simulink model "Last_version_po_STO"  (R2018b)
settings: Solver=FixedStepAuto  StartTime=0.0  StopTime=inf  FixedStep=1e-3  MaxStep=1e-4  RelTol=1e-3
undefined symbols (not defined in the file or in its folder): D11, Delta
libraries: powerlib x118, simulink_extras x25, powerlib_meascontrol x18, simulink x8, xpcutilitieslib x2, xpcrtudplib x2, opclib x1, sldrtlib x1
(part 1 of 3)
settings Model: Creator=YuORLOV  LastModifiedBy=10
settings DataIOCC: SaveOutput=off  SignalLogging=off  DSMLogging=off  SaveTime=off
settings OptimizationCC: BlockReduction=off
settings DebuggingCC: LibraryContextMissingDiagnostic=none
settings SFSimCC: SimUseLocalCustomCode=off
settings RTWCC: RTWUseLocalCustomCode=off
settings CodeAppCC: StateflowObjectComments=on
settings SimscapeCC: SimscapeNormalizeSystem=off

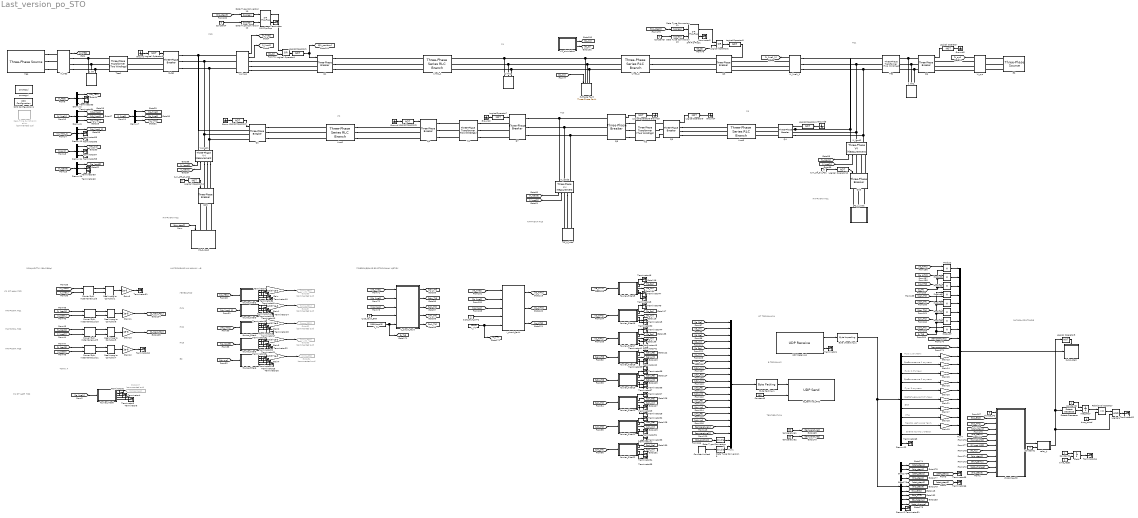
== system Last_version_po_STO ==
  note: ГЕНЕРАТОР
  note: НАПРЯЖЕНИЯ НА ШИНАХ, кВ
  note: ПС2
  note: ПС3
  note: ПС1
  note: ЭС
  note: МОЩНОСТИ, МВт(МВАр)
  note: Л1 ОТ ШИН ПС2
  note: НАГРУЗКА ПС1
  note: НАГРУЗКА ПС2
  note: НАГРУЗКА ПС3
  note: ТОКИ, А
  note: Л1 ОТ ШИН ПС2
  note: НАГРУЗКА ПС3
  note: Л2
  note: Л3
  note: ПС3
  note: ПС1
  note: ПС2
  note: НАГРУЗКА ПС1
  note: НАГРУЗКА ПС2
  note: В ТЕРМИНАЛ
  note: ПОВРЕЖДЕНИЯ ВО ВТОРИЧНЫХ ЦЕПЯХ
  note: ОТ ТЕРМИНАЛА
  note: ЗАПИСЬ COMTRADE
  note: ТЕМПЕРАТУРА
  note: Л1
  note: Пуск 1 ступени
  note: Срабатывание 1 ступени
  note: Пуск 2 ступени
  note: Срабатывание 2 ступени
  note: КТЦ
  note: Неиспр. датчиков темп.
  note: Смена группы уставок
  note: Пуск 3 ступени
  note: Срабатывание 3 ступени
  note: БНН
  1 kW : powerlib/Elements/Three-Phase Parallel RLC Load  LConnTagsString=A|B|C  Configuration=Y (grounded)  NominalVoltage=20e3  Vabc=[1e3 1e3 1e3]  Vabcp=[1e3 1e3 1e3]  NominalFrequency=50  UnbalancedPower=off  ActivePower=1000  InductivePower=0  CapacitivePower=0  Pabc=[10e3 9e3 11e3]  QLabc=[100 90 110]  QCabc=[100 90 110]  Pabcp=[10e3 9e3 11e3]  QLabcp=[100 90 110]  QCabcp=[100 90 110]  Measurements=None  LoadType=constant Z
      settings: SourceProductName=Simscape Electrical
  1 kW1 : powerlib/Elements/Three-Phase Parallel RLC Load  LConnTagsString=A|B|C  Configuration=Y (grounded)  NominalVoltage=20e3  Vabc=[1e3 1e3 1e3]  Vabcp=[1e3 1e3 1e3]  NominalFrequency=50  UnbalancedPower=off  ActivePower=1000  InductivePower=0  CapacitivePower=0  Pabc=[10e3 9e3 11e3]  QLabc=[100 90 110]  QCabc=[100 90 110]  Pabcp=[10e3 9e3 11e3]  QLabcp=[100 90 110]  QCabcp=[100 90 110]  Measurements=None  LoadType=constant Z
      settings: SourceProductName=Simscape Electrical
  1 kW2 : powerlib/Elements/Three-Phase Parallel RLC Load  LConnTagsString=A|B|C  Configuration=Y (grounded)  NominalVoltage=20e3  Vabc=[1e3 1e3 1e3]  Vabcp=[1e3 1e3 1e3]  NominalFrequency=50  UnbalancedPower=off  ActivePower=1000  InductivePower=0  CapacitivePower=0  Pabc=[10e3 9e3 11e3]  QLabc=[100 90 110]  QCabc=[100 90 110]  Pabcp=[10e3 9e3 11e3]  QLabcp=[100 90 110]  QCabcp=[100 90 110]  Measurements=None  LoadType=constant Z
      settings: SourceProductName=Simscape Electrical
  3-Phase Fault : powerlib/Elements/Three-Phase Fault  InitialStates=0  FaultA=on  FaultB=on  FaultC=off  GroundFault=on  SwitchTimes=[ 0.1 0.2]  External=on  SwitchStatus=NaN  FaultResistance=1e-3  GroundResistance=1e-3  SnubberResistance=inf  SnubberCapacitance=inf  Measurements=None
      settings: SourceProductName=Simscape Electrical
  Byte Packing 1 : xpcutilitieslib/Byte Packing   MaskPackedDataType=uint8  MaskUnpackedDataTypes={'double'}  MaskAlignment=1
  Byte Unpacking 1 : xpcutilitieslib/Byte Unpacking   MaskUnpackedDataTypes={'double'}  MaskUnpackedDataSizes={[11]}  MaskAlignment=1
      settings: SourceProductName=Simulink Real-Time  SourceProductBaseCode=XP
  Clock : Integrator  ExternalReset=either
  Constant1 : Constant  Value=4
  Constant2 : Constant
  Constant3 : Constant  Value=160  OutDataTypeStr=double
  Constant4 : Constant  Value=0
  Constant5 : Constant  Value=0
  Constant8 : Constant
  Counter Limited : simulink/Sources/Counter Limited  uplimit=3999  tsamp=-1
  Data Type Conversion{10..13} (4 alike) : DataTypeConversion  OutDataTypeStr=boolean
  Data Type Conversion8 : DataTypeConversion  OutDataTypeStr=double
  Data Type Conversion9 : DataTypeConversion  OutDataTypeStr=double
  Demux{2,6..7,10,14,16} (6 alike) : Demux  Outputs=3
  Demux22 : Demux  Outputs=11
  Demux23 : Demux  Outputs=11
  Detect Decrease : simulink/Logic and Bit Operations/Detect Decrease  vinit=0.0  OutDataTypeStr=boolean
  ES : powerlib/Electrical Sources/Three-Phase Source  InternalConnection=Y  VoltagePhases=off  Voltage=11200  PhaseAngle=0  Voltage_phases=[25e3 25e3 25e3]/sqrt(3)  PhaseAngles_phases=[0 -120 +120]  Frequency=50  NonIdealSource=on  SpecifyImpedance=on  Resistance=0.8929  Inductance=16.58e-3  ShortCircuitLevel=100e12  BaseVoltage=330e3  XRratio=999  BusType=swing  Pref=10e3  Qref=0  Prefabc=[10e3, 10e3, 10e3]  Qrefabc=[0, 0, 0]  Qmin=-inf  Qmax=inf
      settings: SourceProductName=Simscape Electrical
  Gain{,1..4} (5 alike) : Gain  Gain=sqrt(3)*1e-3
  Gain{6,10..12} (4 alike) : Gain  Gain=1e-6
  Gain{13..21} (9 alike) : Gain
  Goto107 : Goto  Commented=on  GotoTag=Irms_line1
  Goto80 : Goto  Commented=on  GotoTag=Vrms_TES
  Goto81 : Goto  Commented=on  GotoTag=Vrms_PS1
  Goto82 : Goto  Commented=on  GotoTag=Vrms_PS2
  Goto83 : Goto  Commented=on  GotoTag=Vrms_PS3
  Goto84 : Goto  Commented=on  GotoTag=Vrms_ES
  Ground{,1..7} (8 alike) : Ground
  I_circuit_fault : Subsystem
  Integrator : Integrator  ExternalReset=rising
  KZ_simulation : Subsystem
  Line1_1 : powerlib/Elements/Three-Phase Series RLC Branch  LConnTagsString=A|B|C  RConnTagsString=A|B|C  BranchType=RLC  Resistance=0.5*7.5  Inductance=0.5*120/(2*pi*50)  Capacitance=0.5*335/(2*pi*50)  Measurements=None
      settings: SourceProductName=Simscape Electrical
  Line1_2 : powerlib/Elements/Three-Phase Series RLC Branch  LConnTagsString=A|B|C  RConnTagsString=A|B|C  BranchType=RLC  Resistance=0.5*7.5  Inductance=0.5*120/(2*pi*50)  Capacitance=0.5*335/(2*pi*50)  Measurements=None
      settings: SourceProductName=Simscape Electrical
  Line2 : powerlib/Elements/Three-Phase Series RLC Branch  LConnTagsString=A|B|C  RConnTagsString=A|B|C  BranchType=RLC  Resistance=1.05  Inductance=16.25/(2*pi*50)  Capacitance=167.5/(2*pi*50)  Measurements=None
      settings: SourceProductName=Simscape Electrical
  Line3 : powerlib/Elements/Three-Phase Series RLC Branch  LConnTagsString=A|B|C  RConnTagsString=A|B|C  BranchType=RLC  Resistance=1.05  Inductance=16.25/(2*pi*50)  Capacitance=167.5/(2*pi*50)  Measurements=None
      settings: SourceProductName=Simscape Electrical
  Logical Operator{,5,11..12} (4 alike) : Logic  Operator=NOT  AllPortsSameDT=off  OutDataTypeStr=boolean
  Logical Operator1 : Logic  Operator=OR  AllPortsSameDT=off  OutDataTypeStr=boolean
  Logical Operator2 : Logic  Operator=OR  AllPortsSameDT=off  OutDataTypeStr=boolean
  Logical Operator3 : Logic  Operator=NOT  Inputs=6  AllPortsSameDT=off  OutDataTypeStr=boolean
  Logical6 : Logic  AllPortsSameDT=off  OutDataTypeStr=boolean
  LogicalOperator{1..4,6..9} (8 alike) : Logic  Operator=NOT  AllPortsSameDT=off  OutDataTypeStr=boolean
  Mux1 : Mux  Inputs=20
  Mux4 : Mux  Inputs=20
  OPC Configuration1 : opclib/OPC Configuration  errMissingItems=Error  errReadWrite=Warn  errShutdown=Error  errRTViolation=Warn  rtEnable=on  speedup=1  showLatency=off  beingUsed=on
      settings: SourceProductName=OPC Toolbox  SourceProductBaseCode=OT
  PS_1_load : Subsystem
  PS_2_load : Subsystem
  PS_3_load : Subsystem
  Power (3ph, Instantaneous){5,9..11} (4 alike) : powerlib_meascontrol/Measurements/Power (3ph, Instantaneous)
      settings: SourceProductName=Simscape Electrical
  Product{,1..7} (8 alike) : Product
  Q{1..9,25..26} (11 alike) : powerlib/Elements/Three-Phase Breaker  InitialState=closed  SwitchA=on  SwitchB=on  SwitchC=on  SwitchTimes="[1/60  5/60]"  External=on  BreakerResistance=0.01  SnubberResistance=1e6  SnubberCapacitance=inf  Measurements=None
      settings: SourceProductName=Simscape Electrical
  Q_tes : powerlib/Elements/Three-Phase Breaker  InitialState=closed  SwitchA=on  SwitchB=on  SwitchC=on  SwitchTimes="[1/60  5/60]"  External=on  BreakerResistance=0.01  SnubberResistance=1e6  SnubberCapacitance=inf  Measurements=None
      settings: SourceProductName=Simscape Electrical
  Real-Imag to Complex{1,5..7} (4 alike) : RealImagToComplex
  Real-Time Synchronization : sldrtlib/Real-Time Synchronization  Commented=on  SampleTime=0.1  MaxMissedTicks=10  ShowMissedTicks=off  YieldWhenWaiting=off
  Relational Operator : RelationalOperator  OutDataTypeStr=boolean  RndMeth=Simplest
  S-R Flip-Flop : simulink_extras/Flip Flops/S-R Flip-Flop  initial_condition=0
  S-R Flip-Flop1 : simulink_extras/Flip Flops/S-R Flip-Flop  initial_condition=0
  Subsystem : Subsystem
  TES : powerlib/Electrical Sources/Three-Phase Source  InternalConnection=Y  VoltagePhases=off  Voltage=19200  PhaseAngle=0  Voltage_phases=[25e3 25e3 25e3]/sqrt(3)  PhaseAngles_phases=[0 -120 +120]  Frequency=50  NonIdealSource=on  SpecifyImpedance=on  Resistance=0.8929  Inductance=16.58e-3  ShortCircuitLevel=100e12  BaseVoltage=330e3  XRratio=999  BusType=swing  Pref=10e3  Qref=0  Prefabc=[10e3, 10e3, 10e3]  Qrefabc=[0, 0, 0]  Qmin=-inf  Qmax=inf
      settings: SourceProductName=Simscape Electrical
  Terminator{,1..66} (67 alike) : Terminator
  Tes : powerlib/Elements/Three-Phase Transformer (Two Windings)  Winding1Connection=Yg  Winding2Connection=Delta (D11)  CoreType=Three single-phase transformers  SetSaturation=off  Hysteresis=off  DataFile='hysteresis'  SetInitialFlux=off  Measurements=None  UNITS=pu  NominalPower=[ 16500e6 , 50 ]  Winding1=[ 330e3 , 0.0005 , 0.189 ]  Winding2=[ 10.5e3 , 0.0005 , 0.189 ]  Rm=500  Lm=500  L0=0.5  Saturation=[ 0,0 ; 0.0024,1.2 ; 1.0,1.52 ]  InitialFluxes=[ 0.8 , -0.8 , 0.7 ]  MoreParameters=off  BreakLoop=off  DataType=off  TransfoNumber=1
      settings: SourceProductName=Simscape Electrical
  Tl2 : powerlib/Elements/Three-Phase Transformer (Two Windings)  Winding1Connection=Yg  Winding2Connection=Yg  CoreType=Three single-phase transformers  SetSaturation=off  Hysteresis=off  DataFile='hysteresis'  SetInitialFlux=off  Measurements=None  UNITS=pu  NominalPower=[ 100e6 , 50 ]  Winding1=[ 330e3 , 0 , 0.05 ]  Winding2=[ 110e3 , 0 , 0.05 ]  Rm=500  Lm=500  L0=0.5  Saturation=[ 0,0 ; 0.0024,1.2 ; 1.0,1.52 ]  InitialFluxes=[ 0.8 , -0.8 , 0.7 ]  MoreParameters=off  BreakLoop=off  DataType=off  TransfoNumber=1
      settings: SourceProductName=Simscape Electrical
  Tl3 : powerlib/Elements/Three-Phase Transformer (Two Windings)  Winding1Connection=Yg  Winding2Connection=Yg  CoreType=Three single-phase transformers  SetSaturation=off  Hysteresis=off  DataFile='hysteresis'  SetInitialFlux=off  Measurements=None  UNITS=pu  NominalPower=[ 100e6 , 50 ]  Winding1=[ 330e3 , 0 , 0.05 ]  Winding2=[ 110e3 , 0 , 0.05 ]  Rm=500  Lm=500  L0=0.5  Saturation=[ 0,0 ; 0.0024,1.2 ; 1.0,1.52 ]  InitialFluxes=[ 0.8 , -0.8 , 0.7 ]  MoreParameters=off  BreakLoop=off  DataType=off  TransfoNumber=1
      settings: SourceProductName=Simscape Electrical
  Ttes1 : powerlib/Elements/Three-Phase Transformer (Two Windings)  Winding1Connection=Yg  Winding2Connection=Delta (D11)  CoreType=Three single-phase transformers  SetSaturation=off  Hysteresis=off  DataFile='hysteresis'  SetInitialFlux=off  Measurements=None  UNITS=SI  NominalPower=[ 630000000, 50]  Winding1=[347000 0.19719 0.034976]  Winding2=[20000 0.00065508 0.00023238]  Rm=10029.9042  Lm=170.8631  L0=0.27511  Saturation=[0 0;3.741 1029.2;1558.8 1303.7]  InitialFluxes=[686.13 -686.13 600.37]  MoreParameters=off  BreakLoop=off  DataType=on  TransfoNumber=1
      settings: SourceProductName=Simscape Electrical
  UDP Receive1 : xpcrtudplib/UDP Receive  ipAddressVal=Use host-target connection  localPort=8002  rcvWidth=88  rcvFmAny=off  fmAddress=192.168.1.250  rcvMulticast=off  multicastAddress=[]  maxUDPQueue=8  sampleTime=1e-3
      settings: SourceProductName=Simulink Real-Time
  U_circuit_fault : Subsystem
  VI_TES : powerlib/Measurements/Three-Phase V-I Measurement  VoltageMeasurement=phase-to-ground  SetLabelV=off  LabelV=V_TES  Vpu=off  VpuLL=off  CurrentMeasurement=no  SetLabelI=off  LabelI=Iabc  Ipu=off  Pbase=100e6  Vbase=500e3  OutputType=Complex  PhasorSimulation=off  PSBequivalent=0
      settings: SourceProductName=Simscape Electrical
  VI_line1 : powerlib/Measurements/Three-Phase V-I Measurement  VoltageMeasurement=phase-to-ground  SetLabelV=off  LabelV=Vabc  Vpu=off  VpuLL=off  CurrentMeasurement=yes  SetLabelI=off  LabelI=Iabc  Ipu=off  Pbase=100e6  Vbase=500e3  OutputType=Complex  PhasorSimulation=off  PSBequivalent=0
      settings: SourceProductName=Simscape Electrical
  VI_line1_1 : powerlib/Measurements/Three-Phase V-I Measurement  VoltageMeasurement=phase-to-ground  SetLabelV=off  LabelV=Vabc  Vpu=off  VpuLL=off  CurrentMeasurement=no  SetLabelI=off  LabelI=Iabc  Ipu=off  Pbase=100e6  Vbase=500e3  OutputType=Complex  PhasorSimulation=off  PSBequivalent=0
      settings: SourceProductName=Simscape Electrical
  VI_load1 : powerlib/Measurements/Three-Phase V-I Measurement  VoltageMeasurement=phase-to-ground  SetLabelV=off  LabelV=Vabc  Vpu=off  VpuLL=off  CurrentMeasurement=yes  SetLabelI=off  LabelI=Iabc  Ipu=off  Pbase=100e6  Vbase=500e3  OutputType=Complex  PhasorSimulation=off  PSBequivalent=0
      settings: SourceProductName=Simscape Electrical
  VI_load2 : powerlib/Measurements/Three-Phase V-I Measurement  VoltageMeasurement=phase-to-ground  SetLabelV=off  LabelV=Vabc  Vpu=off  VpuLL=off  CurrentMeasurement=yes  SetLabelI=off  LabelI=Iabc  Ipu=off  Pbase=100e6  Vbase=500e3  OutputType=Complex  PhasorSimulation=off  PSBequivalent=0
      settings: SourceProductName=Simscape Electrical
  VI_load3 : powerlib/Measurements/Three-Phase V-I Measurement  VoltageMeasurement=phase-to-ground  SetLabelV=off  LabelV=Vabc  Vpu=off  VpuLL=off  CurrentMeasurement=yes  SetLabelI=off  LabelI=Iabc  Ipu=off  Pbase=100e6  Vbase=500e3  OutputType=Complex  PhasorSimulation=off  PSBequivalent=0
      settings: SourceProductName=Simscape Electrical
  VI_sys : powerlib/Measurements/Three-Phase V-I Measurement  VoltageMeasurement=phase-to-ground  SetLabelV=off  LabelV=Vabc  Vpu=off  VpuLL=off  CurrentMeasurement=no  SetLabelI=off  LabelI=Iabc  Ipu=off  Pbase=100e6  Vbase=500e3  OutputType=Complex  PhasorSimulation=off  PSBequivalent=0
      settings: SourceProductName=Simscape Electrical
  choose_PO : Constant  Value=5
  choosing_PO : Subsystem
  fourier_filter15 : Subsystem
  fourier_filter16 : Subsystem
  fourier_filter17 : Subsystem
  fourier_filter18 : Subsystem
  fourier_filter19 : Subsystem
  fourier_filter2 : Subsystem
  fourier_filter20 : Subsystem
  fourier_filter21 : Subsystem
  fourier_filter22 : Subsystem
  fourier_filter3 : Subsystem
  fourier_filter4 : Subsystem
  fourier_filter5 : Subsystem
  fourier_filter6 : Subsystem
  fourier_filter8 : Subsystem
  k_TN : Constant  Value=3300/sqrt(3)
  k_TT : Constant  Value=100/5
  powergui : powerlib/powergui  Priority=2  SimulationMode=Discrete  SampleTime=1e-3  frequency=60  Iterations=50  frequencyindice=50  Pbase=100e6  ErrMax=0.0001  UnitsV=kV  UnitsW=MW  buscounter=0  FunctionMessages=off  echomessages=off  EnableUseOfTLC=off  CurrentSourceSwitches=off  DisableSnubberDevices=off  DisableRonSwitches=off  DisableVfSwitches=off  DisplayEquations=off  SolverType=Tustin/Backward Euler (TBE)  Interpol=off  ExternalGateDelay=off  methode=off  Ts=100  x0status=blocks  SPID=off  SwTol=0  HookPort=off  RestoreLinks=warning  ResistiveCurrentMeasurement=off  Frange=logspace(0,3,50)  Ylog=off  Xlog=off  ShowGrid=off  save=off  variable=ZData  structure=0  ZoomFFT=on  StartTime=0.0  cycles=2  DisplayStyle=off  fundamental=60  FreqAxis=off  MaxFrequency=1000  frequencyindicesteady=1  RmsSteady=1  display=off
  relay_t : Subsystem
  temperature1 : Constant  Value=35  OutDataTypeStr=double
  temperature2 : Constant  Value=35  OutDataTypeStr=double
  time_cmtrd : Constant  Value=6
  time_reset : Constant
  to_terminal_RMS : xpcrtudplib/UDP Send  ipAddressVal=Use host-target connection  localPort=8001  toAddress=192.168.1.250  toPort=25001  sampleTime=1e-3
      settings: SourceProductName=Simulink Real-Time  SourceProductBaseCode=XP
  turn_off_all_PS1 : Constant  Value=0
  turn_off_all_PS2 : Constant  Value=0
  type_fault_BNN : Constant  Value=8
  type_fault_KITC : Constant
  wires:
  Logical Operator/1 -> Q6/1
  LogicalOperator1/1 -> [Q1_position], Q1/1
  LogicalOperator2/1 -> Q2/1
  LogicalOperator3/1 -> Q3/1
  LogicalOperator4/1 -> Q4/1
  VI_TES/1 -> [V_TES]
  VI_line1/2 -> [I_line1]
  VI_line1/1 -> [V_line1]
  VI_line1_1/1 -> [V_line1_1]
  VI_sys/1 -> [V_sys]
  [V_TES] -> Demux2/1
  [V_line1] -> Demux6/1
  [I_line1] -> Demux7/1
  [V_line1_1] -> Demux10/1
  [V_sys] -> Demux14/1
  Demux2/1 -> [Va_TES]
  Demux6/2 -> [Vb_line1]
  Demux6/1 -> [Va_line1]
  Demux6/3 -> [Vc_line1]
  Demux7/3 -> [Ic_line1]
  Demux7/1 -> [Ia_line1]
  Demux7/2 -> [Ib_line1]
  Demux10/1 -> [Va_line1_1]
  Demux14/1 -> [Va_sys]
  Logical Operator5/1 -> Q_tes/1
  VI_load1/1 -> [V_load2]
  VI_load1/2 -> [I_load2]
  VI_load2/2 -> [I_load1]
  VI_load2/1 -> [V_load1]
  VI_load3/1 -> [V_load3]
  VI_load3/2 -> [I_load3]
  Demux16/1 -> [Va_load3]
  [V_load3] -> Demux16/1
  [Va_TES] -> fourier_filter2/1(In1)
  [Va_line1_1] -> fourier_filter3/1(In1)
  [Va_line1] -> fourier_filter4/1(In1)
  [Va_load3] -> fourier_filter5/1(In1)
  [Va_sys] -> fourier_filter6/1(In1)
  fourier_filter2/1(RMS) -> Gain/1
  fourier_filter3/1(RMS) -> Gain1/1
  fourier_filter4/1(RMS) -> Gain2/1
  fourier_filter5/1(RMS) -> Gain3/1
  fourier_filter6/1(RMS) -> Gain4/1
  "Power (3ph, Instantaneous)5"/2 -> Real-Imag to Complex1/2
  [V_line1] -> "Power (3ph, Instantaneous)5"/1
  Real-Imag to Complex1/1 -> Gain6/1
  [I_line1] -> "Power (3ph, Instantaneous)5"/2
  "Power (3ph, Instantaneous)5"/1 -> Real-Imag to Complex1/1
  "Power (3ph, Instantaneous)9"/2 -> Real-Imag to Complex5/2
  [V_load2] -> "Power (3ph, Instantaneous)9"/1
  Real-Imag to Complex5/1 -> Gain10/1
  [I_load2] -> "Power (3ph, Instantaneous)9"/2
  "Power (3ph, Instantaneous)9"/1 -> Real-Imag to Complex5/1
  "Power (3ph, Instantaneous)10"/2 -> Real-Imag to Complex6/2
  [V_load1] -> "Power (3ph, Instantaneous)10"/1
  Real-Imag to Complex6/1 -> Gain11/1
  [I_load1] -> "Power (3ph, Instantaneous)10"/2
  "Power (3ph, Instantaneous)10"/1 -> Real-Imag to Complex6/1
  "Power (3ph, Instantaneous)11"/2 -> Real-Imag to Complex7/2
  [V_load3] -> "Power (3ph, Instantaneous)11"/1
  Real-Imag to Complex7/1 -> Gain12/1
  [I_load3] -> "Power (3ph, Instantaneous)11"/2
  "Power (3ph, Instantaneous)11"/1 -> Real-Imag to Complex7/1
  [Ia_line1] -> fourier_filter8/1(In1)
  LogicalOperator6/1 -> Q5/1
  LogicalOperator7/1 -> Q7/1
  LogicalOperator8/1 -> Q8/1
  LogicalOperator9/1 -> Q9/1
  type_fault_BNN/1 -> U_circuit_fault/4(type_fault)
  [Va_line1] -> U_circuit_fault/1(Ua)
  [Vb_line1] -> U_circuit_fault/2(Ub)
  [Vc_line1] -> U_circuit_fault/3(Uc)
  U_circuit_fault/1(U_an) -> [Uan_TN]
  U_circuit_fault/2(U_bn) -> [Ubn_TN]
  U_circuit_fault/3(U_cn) -> [Ucn_TN]
  U_circuit_fault/4(U_ni) -> [Uni_TN]
  U_circuit_fault/5(U_nk) -> [Unk_TN]
  Logical Operator11/1 -> Q25/1
  turn_off_all_PS2/1 -> Logical Operator11/1
  Logical Operator12/1 -> Q26/1
  turn_off_all_PS1/1 -> Logical Operator12/1
  KZ_simulation/1(to_KZ) -> [to_KZ]
  KZ_simulation/2(to_Q) -> [to_Q]
  [to_KZ] -> 3-Phase Fault/1
  Gain/1 -> Goto80/1
  Gain1/1 -> Goto81/1
  Gain2/1 -> Goto82/1
  Gain3/1 -> Goto83/1
  Gain4/1 -> Goto84/1
  Gain11/1 -> [S_load_PS1]
  Gain10/1 -> [S_load_PS2]
  fourier_filter8/1(RMS) -> Goto107/1
  [to_Q] -> Logical Operator1/2
  Logical Operator1/1 -> LogicalOperator1/1
  [Ia_line1] -> I_circuit_fault/1(Ia_line1)
  [Ib_line1] -> I_circuit_fault/2(Ib_line1)
  [Ic_line1] -> I_circuit_fault/3(Ic_line1)
  type_fault_KITC/1 -> I_circuit_fault/4(type_fault)
  k_TT/1 -> [k_TT], I_circuit_fault/5(k_TT)
  I_circuit_fault/1(Ia_KITC) -> [Ia_KITC]
  I_circuit_fault/3(Ic_KITC) -> [Ic_KITC]
  I_circuit_fault/2(Ib_KITC) -> [Ib_KITC]
  [Ia_KITC] -> fourier_filter15/1(In1)
  [Ib_KITC] -> fourier_filter16/1(In1)
  [Ic_KITC] -> fourier_filter17/1(In1)
  [Uan_TN] -> fourier_filter18/1(In1)
  [Ubn_TN] -> fourier_filter19/1(In1)
  [Ucn_TN] -> fourier_filter20/1(In1)
  [Uni_TN] -> fourier_filter21/1(In1)
  [Unk_TN] -> fourier_filter22/1(In1)
  fourier_filter18/2(Real) -> [Uan_Re]
  fourier_filter18/3(Imag) -> [Uan_Im]
  fourier_filter19/3(Imag) -> [Ubn_Im]
  fourier_filter19/2(Real) -> [Ubn_Re]
  fourier_filter20/3(Imag) -> [Ucn_Im]
  fourier_filter20/2(Real) -> [Ucn_Re]
  fourier_filter21/3(Imag) -> [Uni_Im]
  fourier_filter21/2(Real) -> [Uni_Re]
  fourier_filter22/3(Imag) -> [Unk_Im]
  fourier_filter22/2(Real) -> [Unk_Re]
  fourier_filter15/2(Real) -> [Ia_Re]
  fourier_filter15/3(Imag) -> [Ia_Im]
  fourier_filter16/3(Imag) -> [Ib_Im]
  fourier_filter16/2(Real) -> [Ib_Re]
  fourier_filter17/2(Real) -> [Ic_Re]
  fourier_filter17/3(Imag) -> [Ic_Im]
  [temperature1] -> Mux1/17
  [temperature2] -> Mux1/18
  [Unk_Re] -> Mux1/15
  [Unk_Im] -> Mux1/16
  [Ia_Re] -> Mux1/1
  [Uni_Im] -> Mux1/14
  [Uni_Re] -> Mux1/13
  [Ucn_Im] -> Mux1/12
  [Ucn_Re] -> Mux1/11
  [Ia_Im] -> Mux1/2
  [Ib_Re] -> Mux1/3
  [Ubn_Im] -> Mux1/10
  [Ubn_Re] -> Mux1/9
  [Uan_Im] -> Mux1/8
  [Ib_Im] -> Mux1/4
  [Uan_Re] -> Mux1/7
  [Ic_Re] -> Mux1/5
  [Ic_Im] -> Mux1/6
  Mux4/1 -> Subsystem/1(In1)
  relay_t/1(Out) -> Logical6/2, Detect Decrease/1, Logical Operator3/1
  Constant1/1 -> relay_t/2(t_vv)
  Logical Operator3/1 -> Subsystem/Enable
  k_TN/1 -> [k_TN], U_circuit_fault/5(Kt_TN)
  Product/1 -> Mux4/1
  Product1/1 -> Mux4/2
  Product2/1 -> Mux4/3
  [Ia_KITC] -> Product/1
  [Ib_KITC] -> Product1/1
  [Ic_KITC] -> Product2/1
  [k_TT] -> Product2/2, Product1/2, Product/2
  Product4/1 -> Mux4/5
  Product5/1 -> Mux4/6
  Product6/1 -> Mux4/7
  Product7/1 -> Mux4/8
  [Unk_TN] -> Product7/1
  [Uni_TN] -> Product6/1
  [Ucn_TN] -> Product5/1
  [Ubn_TN] -> Product4/1
  [Uan_TN] -> Product3/2
  [k_TN] -> Product7/2, Product6/2, Product5/2, Product4/2, Product3/1
  Constant3/1 -> to_terminal_RMS/2
  Byte Packing 1/1 -> to_terminal_RMS/1
  Mux1/1 -> Byte Packing 1/1
  UDP Receive1/1 -> Byte Unpacking 1/1
  UDP Receive1/2 -> Terminator1/1
  Byte Unpacking 1/1 -> Demux23/1, Demux22/1
  [Q1_position] -> Data Type Conversion8/1
  Data Type Conversion8/1 -> Mux1/19
  Counter Limited/1 -> Data Type Conversion9/1
  Data Type Conversion9/1 -> Mux1/20
  Product3/1 -> Mux4/4
  [temperature1] -> Mux4/9
  [temperature2] -> Mux4/10
  temperature1/1 -> [temperature1]
  temperature2/1 -> [temperature2]
  Detect Decrease/1 -> Integrator/2
  Constant8/1 -> Integrator/1
  Integrator/1 -> Relational Operator/1
  time_cmtrd/1 -> Relational Operator/2
  Relational Operator/1 -> Logical6/1
  choosing_PO/1(stop_cmtrd) -> relay_t/1(In)
  [trip_BNN] -> choosing_PO/2(trip_BNN)
  [trip_KTC] -> choosing_PO/3(trip_KTC)
  [trip_step1] -> choosing_PO/5(trip_step1)
  [sets_change] -> choosing_PO/11(sets_change)
  [fault_temp] -> choosing_PO/10(fault_temp)
  [trip_step2] -> choosing_PO/9(trip_step2)
  [start_step1] -> choosing_PO/4(start_step1)
  choose_PO/1 -> choosing_PO/1(choose_PO)
  [S_load_PS1] -> choosing_PO/6(S_load_PS1)
  [S_load_PS2] -> choosing_PO/7(S_load_PS2)
  [to_KZ] -> choosing_PO/8(to_KZ)
  Logical Operator2/1 -> LogicalOperator3/1
  [to_Q] -> Logical Operator2/2
  S-R Flip-Flop/1 -> Logical Operator1/1
  [trip_step3] -> Data Type Conversion10/1
  [trip_step3] -> Data Type Conversion11/1
  S-R Flip-Flop1/1 -> Logical Operator2/1
  Data Type Conversion10/1 -> S-R Flip-Flop/1
  Data Type Conversion11/1 -> S-R Flip-Flop1/1
  Constant4/1 -> Data Type Conversion12/1
  Data Type Conversion12/1 -> S-R Flip-Flop/2
  Constant5/1 -> Data Type Conversion13/1
  Data Type Conversion13/1 -> S-R Flip-Flop1/2
  S-R Flip-Flop/2 -> Terminator/1
  S-R Flip-Flop1/2 -> Terminator2/1
  fourier_filter8/2(Real) -> Terminator3/1
  fourier_filter8/3(Imag) -> Terminator4/1
  fourier_filter8/4(Complex) -> Terminator5/1
  fourier_filter8/5(Phase) -> Terminator6/1
  fourier_filter2/2(Real) -> Terminator7/1
  fourier_filter2/3(Imag) -> Terminator8/1
  fourier_filter2/5(Phase) -> Terminator10/1
  fourier_filter2/4(Complex) -> Terminator9/1
  fourier_filter3/2(Real) -> Terminator11/1
  fourier_filter3/3(Imag) -> Terminator12/1
  fourier_filter3/4(Complex) -> Terminator13/1
  fourier_filter3/5(Phase) -> Terminator14/1
  fourier_filter4/2(Real) -> Terminator15/1
  fourier_filter4/3(Imag) -> Terminator16/1
  fourier_filter4/4(Complex) -> Terminator17/1
  fourier_filter4/5(Phase) -> Terminator18/1
  fourier_filter5/2(Real) -> Terminator19/1
  fourier_filter5/3(Imag) -> Terminator20/1
  fourier_filter5/4(Complex) -> Terminator21/1
  fourier_filter5/5(Phase) -> Terminator22/1
  fourier_filter6/2(Real) -> Terminator23/1
  fourier_filter6/3(Imag) -> Terminator24/1
  fourier_filter6/4(Complex) -> Terminator25/1
  fourier_filter6/5(Phase) -> Terminator26/1
  fourier_filter20/1(RMS) -> Terminator27/1
  fourier_filter20/5(Phase) -> Terminator28/1
  fourier_filter20/4(Complex) -> Terminator29/1
  fourier_filter21/4(Complex) -> Terminator31/1
  fourier_filter21/5(Phase) -> Terminator30/1
  fourier_filter21/1(RMS) -> Terminator32/1
  fourier_filter22/1(RMS) -> Terminator33/1
  fourier_filter22/4(Complex) -> Terminator34/1
  fourier_filter22/5(Phase) -> Terminator35/1
  fourier_filter19/5(Phase) -> Terminator36/1
  fourier_filter19/4(Complex) -> Terminator37/1
  fourier_filter19/1(RMS) -> Terminator38/1
  fourier_filter18/5(Phase) -> Terminator39/1
  fourier_filter18/4(Complex) -> Terminator40/1
  fourier_filter18/1(RMS) -> Terminator41/1
  fourier_filter17/5(Phase) -> Terminator42/1
  fourier_filter17/4(Complex) -> Terminator43/1
  fourier_filter17/1(RMS) -> Terminator44/1
  fourier_filter16/5(Phase) -> Terminator45/1
  fourier_filter15/1(RMS) -> Terminator46/1
  fourier_filter15/4(Complex) -> Terminator47/1
  fourier_filter15/5(Phase) -> Terminator48/1
  fourier_filter16/1(RMS) -> Terminator49/1
  fourier_filter16/4(Complex) -> Terminator50/1
  Ground/1 -> LogicalOperator2/1
  Ground1/1 -> LogicalOperator6/1
  Ground2/1 -> LogicalOperator7/1
  Ground3/1 -> LogicalOperator8/1
  Ground4/1 -> LogicalOperator9/1
  Ground5/1 -> LogicalOperator4/1
  Ground6/1 -> Logical Operator/1
  Ground7/1 -> Logical Operator5/1
  Logical6/1 -> Terminator52/1
  Demux2/2 -> Terminator53/1
  Demux2/3 -> Terminator54/1
  Demux10/2 -> Terminator55/1
  Demux10/3 -> Terminator56/1
  Demux14/2 -> Terminator57/1
  Demux14/3 -> Terminator58/1
  Demux16/2 -> Terminator59/1
  Demux16/3 -> Terminator60/1
  Gain6/1 -> Terminator61/1
  Gain12/1 -> Terminator62/1
  Gain21/1 -> Mux4/16
  Gain20/1 -> Mux4/15
  Gain17/1 -> Mux4/17
  Gain19/1 -> Mux4/19
  Gain18/1 -> Mux4/18
  Gain16/1 -> Mux4/14
  Gain15/1 -> Mux4/13
  Gain14/1 -> Mux4/12
  Gain13/1 -> Mux4/11
  Demux22/2 -> Gain14/1
  Demux22/1 -> Gain13/1
  Demux22/3 -> Gain15/1
  Demux22/4 -> Gain16/1
  Demux22/5 -> Gain20/1
  Demux22/6 -> Gain21/1
  Demux22/7 -> Gain17/1
  Demux22/8 -> Gain18/1
  Demux22/9 -> Gain19/1
  Demux22/10 -> Mux4/20
  Demux23/6 -> [trip_step3]
  Demux23/5 -> [start_step3]
  Demux23/4 -> [trip_step2]
  Demux23/10 -> [sets_change]
  Demux23/9 -> [fault_temp]
  Demux23/8 -> [trip_KTC]
  Demux23/7 -> [trip_BNN]
  Demux23/3 -> [start_step2]
  Demux23/2 -> [trip_step1]
  Demux23/1 -> [start_step1]
  Demux23/11 -> Terminator51/1
  [trip_step2] -> PS_2_load/1(trip_step2)
  [trip_step3] -> choosing_PO/12(trip_step3)
  Constant2/1 -> Clock/1
  time_reset/1 -> Clock/2
  Demux22/11 -> Terminator63/1
  Clock/1 -> Terminator64/1
  [start_step2] -> Terminator65/1
  [start_step3] -> Terminator66/1
  connections:
  Line1_2/LConn1 -- 1 kW1/LConn1 -- Line1_1/RConn1 -- 3-Phase Fault/LConn1
  Line1_2/LConn2 -- 1 kW1/LConn2 -- Line1_1/RConn2 -- 3-Phase Fault/LConn2
  Line1_2/LConn3 -- 1 kW1/LConn3 -- Line1_1/RConn3 -- 3-Phase Fault/LConn3
  Tes/LConn3 -- VI_load2/LConn3 -- Q4/LConn3 -- VI_line1_1/LConn3
  Q6/RConn1 -- 1 kW2/LConn1 -- Tes/RConn1
  Q6/RConn2 -- 1 kW2/LConn2 -- Tes/RConn2
  Q6/RConn3 -- 1 kW2/LConn3 -- Tes/RConn3
  VI_sys/RConn3 -- Q6/LConn3
  VI_sys/RConn2 -- Q6/LConn2
  VI_sys/RConn1 -- Q6/LConn1
  ES/RConn1 -- VI_sys/LConn1
  ES/RConn2 -- VI_sys/LConn2
  ES/RConn3 -- VI_sys/LConn3
  Q1/RConn1 -- Line1_1/LConn1
  Q1/RConn2 -- Line1_1/LConn2
  Q1/RConn3 -- Line1_1/LConn3
  Q2/RConn1 -- Line2/LConn1
  Q2/RConn2 -- Line2/LConn2
  Q2/RConn3 -- Line2/LConn3
  Q3/RConn1 -- Line1_2/RConn1
  Q3/RConn3 -- Line1_2/RConn3
  Q4/RConn1 -- Line3/RConn1
  Q4/RConn2 -- Line3/RConn2
  Q4/RConn3 -- Line3/RConn3
  VI_line1/RConn2 -- Q1/LConn2
  VI_line1/RConn1 -- Q1/LConn1
  VI_line1/RConn3 -- Q1/LConn3
  Line1_2/RConn2 -- Q3/RConn2
  Q_tes/LConn1 -- Ttes1/LConn1
  Q_tes/LConn2 -- Ttes1/LConn2
  Q_tes/LConn3 -- Ttes1/LConn3
  VI_line1/LConn2 -- VI_load1/LConn2 -- Q2/LConn2 -- Q_tes/RConn2
  Q_tes/RConn1 -- VI_load1/LConn1 -- Q2/LConn1 -- VI_line1/LConn1
  VI_line1_1/RConn2 -- Q3/LConn2
  VI_line1_1/RConn1 -- Q3/LConn1
  VI_line1_1/RConn3 -- Q3/LConn3
  Tes/LConn2 -- VI_load2/LConn2 -- Q4/LConn2 -- VI_line1_1/LConn2
  Q4/LConn1 -- VI_line1_1/LConn1 -- Tes/LConn1 -- VI_load2/LConn1
  VI_line1/LConn3 -- VI_load1/LConn3 -- Q2/LConn3 -- Q_tes/RConn3
  VI_load1/RConn2 -- Q25/LConn2
  Q5/RConn1 -- Tl2/LConn1
  Q5/RConn3 -- Tl2/LConn3
  Q5/RConn2 -- Tl2/LConn2
  Line2/RConn1 -- Q5/LConn1
  Line2/RConn2 -- Q5/LConn2
  Line2/RConn3 -- Q5/LConn3
  Tl2/RConn1 -- Q7/LConn1
  Tl2/RConn2 -- Q7/LConn2
  Tl2/RConn3 -- Q7/LConn3
  Q7/RConn1 -- VI_load3/LConn1 -- Q8/RConn1
  Q7/RConn2 -- VI_load3/LConn2 -- Q8/RConn2
  Q7/RConn3 -- VI_load3/LConn3 -- Q8/RConn3
  Q8/LConn1 -- Tl3/RConn1
  Q8/LConn2 -- Tl3/RConn2
  Q8/LConn3 -- Tl3/RConn3
  Q9/RConn2 -- Tl3/LConn2
  Q9/RConn1 -- Tl3/LConn1
  Q9/RConn3 -- Tl3/LConn3
  Q9/LConn1 -- Line3/LConn1
  Q9/LConn2 -- Line3/LConn2
  Q9/LConn3 -- Line3/LConn3
  TES/RConn1 -- VI_TES/LConn1
  TES/RConn2 -- VI_TES/LConn2
  TES/RConn3 -- VI_TES/LConn3
  VI_TES/RConn2 -- 1 kW/LConn2 -- Ttes1/RConn2
  VI_TES/RConn1 -- 1 kW/LConn1 -- Ttes1/RConn1
  VI_TES/RConn3 -- 1 kW/LConn3 -- Ttes1/RConn3
  VI_load1/RConn1 -- Q25/LConn1
  VI_load1/RConn3 -- Q25/LConn3
  Q26/LConn3 -- VI_load2/RConn3
  Q26/LConn2 -- VI_load2/RConn2
  Q26/LConn1 -- VI_load2/RConn1
  PS_2_load/LConn2 -- Q25/RConn2
  PS_2_load/LConn1 -- Q25/RConn1
  PS_2_load/LConn3 -- Q25/RConn3
  PS_3_load/LConn1 -- VI_load3/RConn1
  VI_load3/RConn2 -- PS_3_load/LConn2
  PS_3_load/LConn3 -- VI_load3/RConn3
  PS_1_load/LConn1 -- Q26/RConn1
  PS_1_load/LConn2 -- Q26/RConn2
  PS_1_load/LConn3 -- Q26/RConn3

== system Last_version_po_STO/I_circuit_fault ==
  Ia_line1 : Inport
  Ib_line1 : Inport  Port=2
  Ic_line1 : Inport  Port=3
  type_fault : Inport  Port=4
  k_TT : Inport  Port=5
  Divide : Product  Inputs=*/
  Divide1 : Product  Inputs=*/
  Divide2 : Product  Inputs=*/
  Ground : Ground
  Ground1 : Ground
  Ground2 : Ground
  Multiport Switch : MultiPortSwitch
  Multiport Switch1 : MultiPortSwitch
  Multiport Switch2 : MultiPortSwitch
  Ia_KITC : Outport
  Ib_KITC : Outport  Port=2
  Ic_KITC : Outport  Port=3
  wires:
  Ib_line1/1 -> Divide1/1
  k_TT/1 -> Divide2/2, Divide1/2, Divide/2
  [type_fault] -> Multiport Switch/1
  [type_fault] -> Multiport Switch2/1
  [Ib_line1] -> Multiport Switch1/2
  type_fault/1 -> [type_fault]
  [Ia_line1] -> Multiport Switch/2
  Ia_line1/1 -> Divide/1
  Divide/1 -> [Ia_line1]
  [type_fault] -> Multiport Switch1/1
  Divide2/1 -> [Ic_line1]
  Divide1/1 -> [Ib_line1]
  [Ic_line1] -> Multiport Switch2/2
  Ic_line1/1 -> Divide2/1
  [Ib_line1] -> Multiport Switch1/3
  Multiport Switch1/1 -> Ib_KITC/1
  Multiport Switch2/1 -> Ic_KITC/1
  Multiport Switch/1 -> Ia_KITC/1
  [Ic_line1] -> Multiport Switch2/3
  [Ic_line1] -> Multiport Switch2/4
  Ground/1 -> Multiport Switch/3
  Ground1/1 -> Multiport Switch/4
  Ground2/1 -> Multiport Switch1/4

== system Last_version_po_STO/KZ_simulation ==
  Data Type Conversion : DataTypeConversion  OutDataTypeStr=double
  Logical Operator3 : Logic  Operator=XOR  AllPortsSameDT=off  OutDataTypeStr=boolean
  Logical Operator4 : Logic  Operator=XOR  AllPortsSameDT=off  OutDataTypeStr=boolean
  Logical Operator5 : Logic  Operator=XOR  AllPortsSameDT=off  OutDataTypeStr=boolean
  pause_APV : Constant  Value=3
  relay_t : Subsystem
  relay_t1 : Subsystem
  start_KZ : Constant  Value=0  OutDataTypeStr=boolean
  time_kz : Constant  Value=2
  to_KZ : Outport
  to_Q : Outport  Port=2
  wires:
  Logical Operator4/1 -> Logical Operator5/2
  Logical Operator3/1 -> Logical Operator5/1, Data Type Conversion/1
  relay_t1/1(Out) -> Logical Operator4/2
  time_kz/1 -> relay_t/2(t_vv)
  Logical Operator5/1 -> to_Q/1
  start_KZ/1 -> Logical Operator4/1, relay_t1/1(In), Logical Operator3/1, relay_t/1(In)
  relay_t/1(Out) -> Logical Operator3/2
  pause_APV/1 -> relay_t1/2(t_vv)
  Data Type Conversion/1 -> to_KZ/1

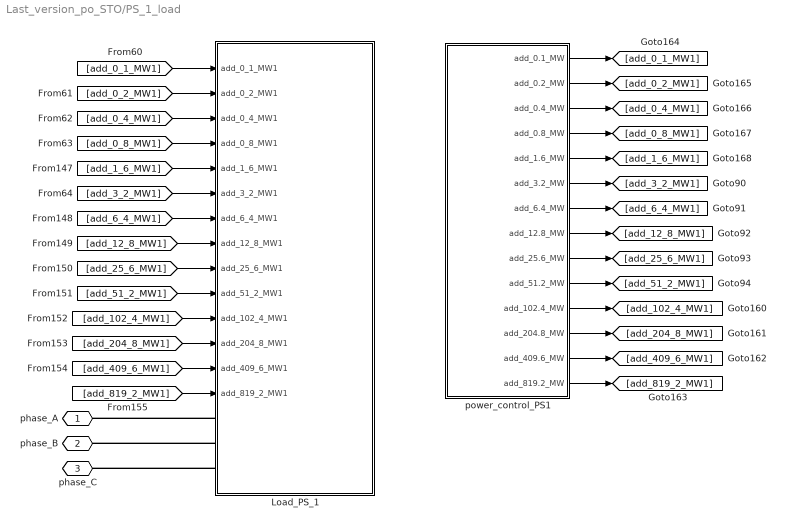
== system Last_version_po_STO/PS_1_load ==
  Load_PS_1 : Subsystem
  power_control_PS1 : Subsystem
  phase_A : PMIOPort  Side=Left
  phase_B : PMIOPort  Port=2  Side=Left
  phase_C : PMIOPort  Port=3  Side=Left
  wires:
  power_control_PS1/7(add_6.4_MW) -> [add_6_4_MW1]
  [add_0_2_MW1] -> Load_PS_1/2(add_0_2_MW1)
  power_control_PS1/14(add_819.2_MW) -> [add_819_2_MW1]
  [add_0_1_MW1] -> Load_PS_1/1(add_0_1_MW1)
  power_control_PS1/4(add_0.8_MW) -> [add_0_8_MW1]
  power_control_PS1/3(add_0.4_MW) -> [add_0_4_MW1]
  [add_409_6_MW1] -> Load_PS_1/13(add_409_6_MW1)
  power_control_PS1/13(add_409.6_MW) -> [add_409_6_MW1]
  power_control_PS1/5(add_1.6_MW) -> [add_1_6_MW1]
  power_control_PS1/8(add_12.8_MW) -> [add_12_8_MW1]
  [add_0_4_MW1] -> Load_PS_1/3(add_0_4_MW1)
  power_control_PS1/10(add_51.2_MW) -> [add_51_2_MW1]
  [add_0_8_MW1] -> Load_PS_1/4(add_0_8_MW1)
  [add_1_6_MW1] -> Load_PS_1/5(add_1_6_MW1)
  power_control_PS1/11(add_102.4_MW) -> [add_102_4_MW1]
  [add_6_4_MW1] -> Load_PS_1/7(add_6_4_MW1)
  [add_12_8_MW1] -> Load_PS_1/8(add_12_8_MW1)
  [add_25_6_MW1] -> Load_PS_1/9(add_25_6_MW1)
  [add_102_4_MW1] -> Load_PS_1/11(add_102_4_MW1)
  power_control_PS1/12(add_204.8_MW) -> [add_204_8_MW1]
  power_control_PS1/1(add_0.1_MW) -> [add_0_1_MW1]
  power_control_PS1/6(add_3.2_MW) -> [add_3_2_MW1]
  [add_204_8_MW1] -> Load_PS_1/12(add_204_8_MW1)
  power_control_PS1/2(add_0.2_MW) -> [add_0_2_MW1]
  power_control_PS1/9(add_25.6_MW) -> [add_25_6_MW1]
  [add_51_2_MW1] -> Load_PS_1/10(add_51_2_MW1)
  [add_3_2_MW1] -> Load_PS_1/6(add_3_2_MW1)
  [add_819_2_MW1] -> Load_PS_1/14(add_819_2_MW1)
  connections:
  Load_PS_1/LConn1 -- phase_A/RConn1
  Load_PS_1/LConn2 -- phase_B/RConn1
  Load_PS_1/LConn3 -- phase_C/RConn1

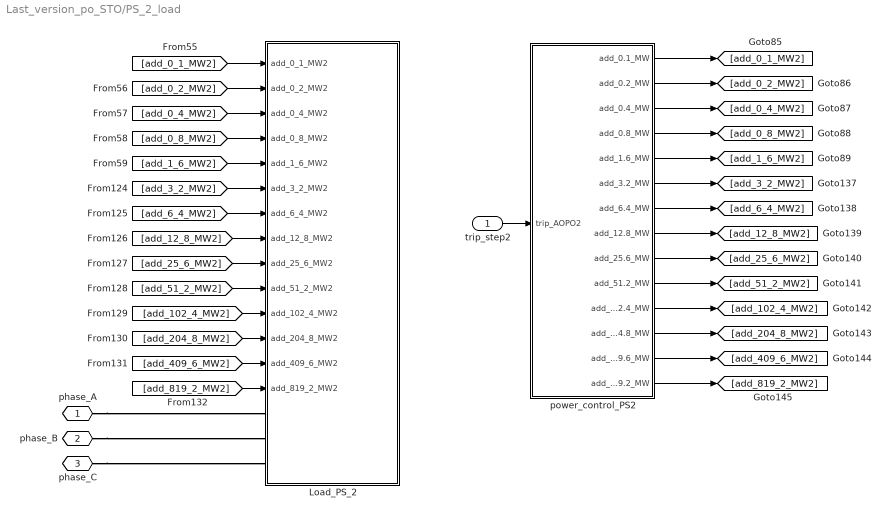
== system Last_version_po_STO/PS_2_load ==
  trip_step2 : Inport
  Load_PS_2 : Subsystem
  power_control_PS2 : Subsystem
  phase_A : PMIOPort  Side=Left
  phase_B : PMIOPort  Port=2  Side=Left
  phase_C : PMIOPort  Port=3  Side=Left
  wires:
  power_control_PS2/3(add_0.4_MW) -> [add_0_4_MW2]
  power_control_PS2/6(add_3.2_MW) -> [add_3_2_MW2]
  power_control_PS2/14(add_819.2_MW) -> [add_819_2_MW2]
  power_control_PS2/2(add_0.2_MW) -> [add_0_2_MW2]
  power_control_PS2/7(add_6.4_MW) -> [add_6_4_MW2]
  power_control_PS2/8(add_12.8_MW) -> [add_12_8_MW2]
  [add_0_1_MW2] -> Load_PS_2/1(add_0_1_MW2)
  [add_1_6_MW2] -> Load_PS_2/5(add_1_6_MW2)
  power_control_PS2/1(add_0.1_MW) -> [add_0_1_MW2]
  [add_12_8_MW2] -> Load_PS_2/8(add_12_8_MW2)
  [add_25_6_MW2] -> Load_PS_2/9(add_25_6_MW2)
  [add_51_2_MW2] -> Load_PS_2/10(add_51_2_MW2)
  [add_102_4_MW2] -> Load_PS_2/11(add_102_4_MW2)
  [add_204_8_MW2] -> Load_PS_2/12(add_204_8_MW2)
  [add_819_2_MW2] -> Load_PS_2/14(add_819_2_MW2)
  power_control_PS2/4(add_0.8_MW) -> [add_0_8_MW2]
  [add_409_6_MW2] -> Load_PS_2/13(add_409_6_MW2)
  power_control_PS2/11(add_102.4_MW) -> [add_102_4_MW2]
  [add_6_4_MW2] -> Load_PS_2/7(add_6_4_MW2)
  [add_0_2_MW2] -> Load_PS_2/2(add_0_2_MW2)
  [add_0_8_MW2] -> Load_PS_2/4(add_0_8_MW2)
  power_control_PS2/13(add_409.6_MW) -> [add_409_6_MW2]
  [add_0_4_MW2] -> Load_PS_2/3(add_0_4_MW2)
  [add_3_2_MW2] -> Load_PS_2/6(add_3_2_MW2)
  power_control_PS2/12(add_204.8_MW) -> [add_204_8_MW2]
  power_control_PS2/9(add_25.6_MW) -> [add_25_6_MW2]
  power_control_PS2/10(add_51.2_MW) -> [add_51_2_MW2]
  power_control_PS2/5(add_1.6_MW) -> [add_1_6_MW2]
  trip_step2/1 -> power_control_PS2/1(trip_AOPO2)
  connections:
  phase_B/RConn1 -- Load_PS_2/LConn2
  phase_A/RConn1 -- Load_PS_2/LConn1
  phase_C/RConn1 -- Load_PS_2/LConn3

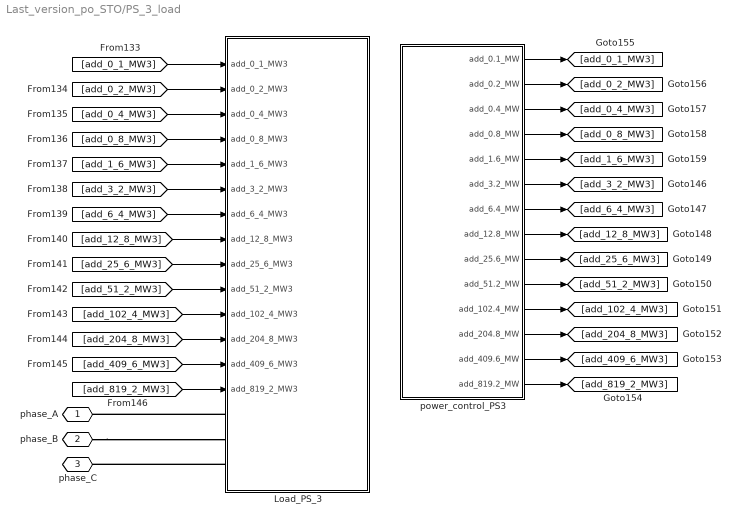
== system Last_version_po_STO/PS_3_load ==
  Load_PS_3 : Subsystem
  power_control_PS3 : Subsystem
  phase_A : PMIOPort  Side=Left
  phase_B : PMIOPort  Port=2  Side=Left
  phase_C : PMIOPort  Port=3  Side=Left
  wires:
  power_control_PS3/6(add_3.2_MW) -> [add_3_2_MW3]
  power_control_PS3/14(add_819.2_MW) -> [add_819_2_MW3]
  [add_0_1_MW3] -> Load_PS_3/1(add_0_1_MW3)
  power_control_PS3/4(add_0.8_MW) -> [add_0_8_MW3]
  power_control_PS3/12(add_204.8_MW) -> [add_204_8_MW3]
  power_control_PS3/11(add_102.4_MW) -> [add_102_4_MW3]
  power_control_PS3/9(add_25.6_MW) -> [add_25_6_MW3]
  power_control_PS3/8(add_12.8_MW) -> [add_12_8_MW3]
  power_control_PS3/3(add_0.4_MW) -> [add_0_4_MW3]
  [add_0_4_MW3] -> Load_PS_3/3(add_0_4_MW3)
  [add_1_6_MW3] -> Load_PS_3/5(add_1_6_MW3)
  [add_12_8_MW3] -> Load_PS_3/8(add_12_8_MW3)
  [add_204_8_MW3] -> Load_PS_3/12(add_204_8_MW3)
  power_control_PS3/7(add_6.4_MW) -> [add_6_4_MW3]
  [add_819_2_MW3] -> Load_PS_3/14(add_819_2_MW3)
  [add_51_2_MW3] -> Load_PS_3/10(add_51_2_MW3)
  [add_0_2_MW3] -> Load_PS_3/2(add_0_2_MW3)
  [add_0_8_MW3] -> Load_PS_3/4(add_0_8_MW3)
  [add_409_6_MW3] -> Load_PS_3/13(add_409_6_MW3)
  power_control_PS3/1(add_0.1_MW) -> [add_0_1_MW3]
  power_control_PS3/13(add_409.6_MW) -> [add_409_6_MW3]
  [add_102_4_MW3] -> Load_PS_3/11(add_102_4_MW3)
  power_control_PS3/10(add_51.2_MW) -> [add_51_2_MW3]
  power_control_PS3/2(add_0.2_MW) -> [add_0_2_MW3]
  power_control_PS3/5(add_1.6_MW) -> [add_1_6_MW3]
  [add_25_6_MW3] -> Load_PS_3/9(add_25_6_MW3)
  [add_6_4_MW3] -> Load_PS_3/7(add_6_4_MW3)
  [add_3_2_MW3] -> Load_PS_3/6(add_3_2_MW3)
  connections:
  phase_B/RConn1 -- Load_PS_3/LConn2
  Load_PS_3/LConn3 -- phase_C/RConn1
  Load_PS_3/LConn1 -- phase_A/RConn1

== system Last_version_po_STO/Subsystem ==
  In1 : Inport
  Enable : EnablePort
  ToWorkspace : ToWorkspace  VariableName=cmtrd_data  SaveFormat=Timeseries  SampleTime=-1
      settings: MaxDataPoints=6000
  wires:
  In1/1 -> ToWorkspace/1

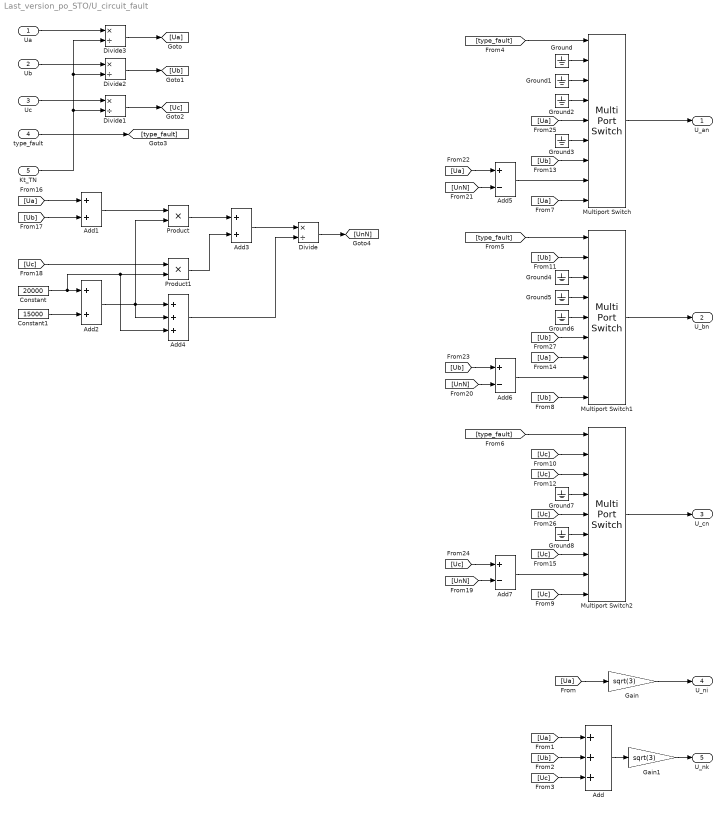
== system Last_version_po_STO/U_circuit_fault ==
  Ua : Inport
  Ub : Inport  Port=2
  Uc : Inport  Port=3
  type_fault : Inport  Port=4
  Kt_TN : Inport  Port=5
  Add : Sum  Inputs=+++
  Add1 : Sum
  Add2 : Sum
  Add3 : Sum
  Add4 : Sum  Inputs=+++
  Add5 : Sum  Inputs=+-
  Add6 : Sum  Inputs=+-
  Add7 : Sum  Inputs=+-
  Constant : Constant  Value=20000
  Constant1 : Constant  Value=15000
  Divide{,1..3} (4 alike) : Product  Inputs=*/
  Gain : Gain  Gain=sqrt(3)
  Gain1 : Gain  Gain=sqrt(3)
  Ground{,1..8} (9 alike) : Ground
  Multiport Switch : MultiPortSwitch  Inputs=8
  Multiport Switch1 : MultiPortSwitch  Inputs=8
  Multiport Switch2 : MultiPortSwitch  Inputs=8
  Product : Product
  Product1 : Product
  U_an : Outport
  U_bn : Outport  Port=2
  U_cn : Outport  Port=3
  U_ni : Outport  Port=4
  U_nk : Outport  Port=5
  wires:
  [Ua] -> Gain/1
  Gain/1 -> U_ni/1
  [Ua] -> Add/1
  [Ub] -> Add/2
  [Uc] -> Add/3
  Add/1 -> Gain1/1
  Gain1/1 -> U_nk/1
  [type_fault] -> Multiport Switch/1
  type_fault/1 -> [type_fault]
  Multiport Switch/1 -> U_an/1
  Multiport Switch1/1 -> U_bn/1
  Multiport Switch2/1 -> U_cn/1
  [type_fault] -> Multiport Switch1/1
  [type_fault] -> Multiport Switch2/1
  [Ua] -> Multiport Switch/9
  [Ub] -> Multiport Switch1/9
  [Uc] -> Multiport Switch2/9
  [Uc] -> Multiport Switch2/2
  [Ub] -> Multiport Switch1/2
  [Uc] -> Multiport Switch2/3
  [Ub] -> Multiport Switch/7
  [Ua] -> Multiport Switch1/7
  [Uc] -> Multiport Switch2/7
  [Ua] -> Add1/1
  [Ub] -> Add1/2
  Add1/1 -> Product/1
  Constant/1 -> Add4/3, Product1/2, Add2/1
  Constant1/1 -> Add2/2
  Add2/1 -> Add4/2, Add4/1, Product/2
  [Uc] -> Product1/1
  Product/1 -> Add3/1
  Product1/1 -> Add3/2
  Add3/1 -> Divide/1
  Add4/1 -> Divide/2
  Divide/1 -> [UnN]
  Add5/1 -> Multiport Switch/8
  Add6/1 -> Multiport Switch1/8
  Add7/1 -> Multiport Switch2/8
  [UnN] -> Add7/2
  [UnN] -> Add6/2
  [UnN] -> Add5/2
  [Ua] -> Add5/1
  [Ub] -> Add6/1
  [Uc] -> Add7/1
  Divide1/1 -> [Uc]
  Kt_TN/1 -> Divide3/2, Divide2/2, Divide1/2
  Uc/1 -> Divide1/1
  Divide2/1 -> [Ub]
  Divide3/1 -> [Ua]
  Ua/1 -> Divide3/1
  Ub/1 -> Divide2/1
  [Ua] -> Multiport Switch/5
  [Uc] -> Multiport Switch2/5
  [Ub] -> Multiport Switch1/6
  Ground/1 -> Multiport Switch/2
  Ground1/1 -> Multiport Switch/3
  Ground2/1 -> Multiport Switch/4
  Ground3/1 -> Multiport Switch/6
  Ground4/1 -> Multiport Switch1/3
  Ground5/1 -> Multiport Switch1/4
  Ground6/1 -> Multiport Switch1/5
  Ground7/1 -> Multiport Switch2/4
  Ground8/1 -> Multiport Switch2/6

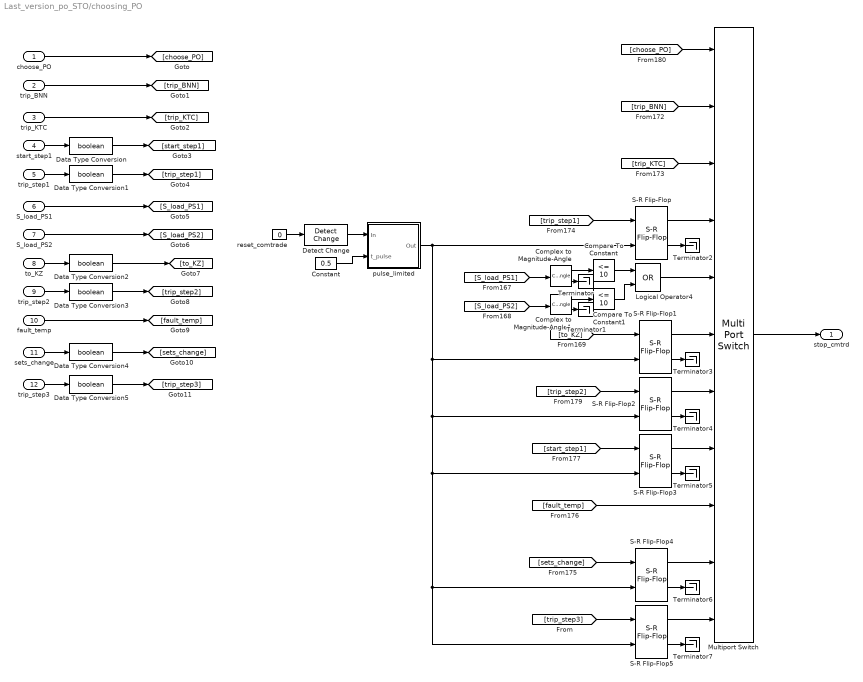
== system Last_version_po_STO/choosing_PO ==
  choose_PO : Inport
  trip_BNN : Inport  Port=2
  trip_KTC : Inport  Port=3
  start_step1 : Inport  Port=4
  trip_step1 : Inport  Port=5
  S_load_PS1 : Inport  Port=6
  S_load_PS2 : Inport  Port=7
  to_KZ : Inport  Port=8
  trip_step2 : Inport  Port=9
  fault_temp : Inport  Port=10
  sets_change : Inport  Port=11
  trip_step3 : Inport  Port=12
  Compare To Constant : simulink/Logic and Bit Operations/Compare To Constant  relop=<=  const=10  OutDataTypeStr=boolean
  Compare To Constant1 : simulink/Logic and Bit Operations/Compare To Constant  relop=<=  const=10  OutDataTypeStr=boolean
  Complex to Magnitude-Angle : ComplexToMagnitudeAngle
  Complex to Magnitude-Angle1 : ComplexToMagnitudeAngle
  Constant : Constant  Value=0.5
  Data Type Conversion{,1..5} (6 alike) : DataTypeConversion  OutDataTypeStr=boolean
  Detect Change : simulink/Logic and Bit Operations/Detect Change  vinit=0  OutDataTypeStr=boolean
  Logical Operator4 : Logic  Operator=OR  AllPortsSameDT=off  OutDataTypeStr=boolean
  Multiport Switch : MultiPortSwitch  Inputs=10
  S-R Flip-Flop{,1..5} (6 alike) : simulink_extras/Flip Flops/S-R Flip-Flop  initial_condition=0
  Terminator{,1..7} (8 alike) : Terminator
  pulse_limited : Subsystem
  reset_comtrade : Constant  Value=0  OutDataTypeStr=boolean
  stop_cmtrd : Outport
  wires:
  Logical Operator4/1 -> Multiport Switch/5
  [trip_KTC] -> Multiport Switch/3
  S-R Flip-Flop3/1 -> Multiport Switch/8
  [trip_step1] -> S-R Flip-Flop/1
  Compare To Constant1/1 -> Logical Operator4/2
  S-R Flip-Flop/1 -> Multiport Switch/4
  [trip_BNN] -> Multiport Switch/2
  Complex to Magnitude-Angle/1 -> Compare To Constant/1
  S-R Flip-Flop4/1 -> Multiport Switch/10
  S-R Flip-Flop2/1 -> Multiport Switch/7
  [fault_temp] -> Multiport Switch/9
  Multiport Switch/1 -> stop_cmtrd/1
  [S_load_PS1] -> Complex to Magnitude-Angle/1
  [S_load_PS2] -> Complex to Magnitude-Angle1/1
  reset_comtrade/1 -> Detect Change/1
  Compare To Constant/1 -> Logical Operator4/1
  [sets_change] -> S-R Flip-Flop4/1
  Complex to Magnitude-Angle1/1 -> Compare To Constant1/1
  [trip_step2] -> S-R Flip-Flop2/1
  [start_step1] -> S-R Flip-Flop3/1
  S-R Flip-Flop1/1 -> Multiport Switch/6
  [choose_PO] -> Multiport Switch/1
  [to_KZ] -> S-R Flip-Flop1/1
  choose_PO/1 -> [choose_PO]
  trip_BNN/1 -> [trip_BNN]
  trip_KTC/1 -> [trip_KTC]
  start_step1/1 -> Data Type Conversion/1
  S_load_PS1/1 -> [S_load_PS1]
  S_load_PS2/1 -> [S_load_PS2]
  to_KZ/1 -> Data Type Conversion2/1
  trip_step2/1 -> Data Type Conversion3/1
  fault_temp/1 -> [fault_temp]
  sets_change/1 -> Data Type Conversion4/1
  trip_step1/1 -> Data Type Conversion1/1
  Complex to Magnitude-Angle/2 -> Terminator/1
  Complex to Magnitude-Angle1/2 -> Terminator1/1
  trip_step3/1 -> Data Type Conversion5/1
  Data Type Conversion/1 -> [start_step1]
  Data Type Conversion1/1 -> [trip_step1]
  Data Type Conversion2/1 -> [to_KZ]
  Data Type Conversion3/1 -> [trip_step2]
  Data Type Conversion4/1 -> [sets_change]
  Data Type Conversion5/1 -> [trip_step3]
  S-R Flip-Flop/2 -> Terminator2/1
  S-R Flip-Flop1/2 -> Terminator3/1
  S-R Flip-Flop2/2 -> Terminator4/1
  S-R Flip-Flop3/2 -> Terminator5/1
  S-R Flip-Flop5/1 -> Multiport Switch/11
  [trip_step3] -> S-R Flip-Flop5/1
  S-R Flip-Flop4/2 -> Terminator6/1
  S-R Flip-Flop5/2 -> Terminator7/1
  Detect Change/1 -> pulse_limited/1(In)
  pulse_limited/1(Out) -> S-R Flip-Flop2/2, S-R Flip-Flop3/2, S-R Flip-Flop4/2, S-R Flip-Flop5/2, S-R Flip-Flop1/2, S-R Flip-Flop/2
  Constant/1 -> pulse_limited/2(t_pulse)

== system Last_version_po_STO/fourier_filter15 ==
  In1 : Inport
  Complex to Real-Imag1 : ComplexToRealImag
  Degrees to Radians : simulink_extras/Transformations/Degrees to Radians
  Fourier1 : powerlib_meascontrol/Measurements/Fourier  Freq=50  n=1  InInit=[0, 0]  Ts=0
      settings: SourceProductName=Simscape Electrical
  Gain1 : Gain  Gain=1/sqrt(2)
  Magnitude-Angle to Complex1 : MagnitudeAngleToComplex
  RMS : Outport
  Real : Outport  Port=2
  Imag : Outport  Port=3
  Complex : Outport  Port=4
  Phase : Outport  Port=5
  wires:
  Gain1/1 -> Magnitude-Angle to Complex1/1, RMS/1
  Fourier1/1 -> Gain1/1
  Degrees to Radians/1 -> Magnitude-Angle to Complex1/2, Phase/1
  Complex to Real-Imag1/1 -> Real/1
  Complex to Real-Imag1/2 -> Imag/1
  Magnitude-Angle to Complex1/1 -> Complex to Real-Imag1/1, Complex/1
  In1/1 -> Fourier1/1
  Fourier1/2 -> Degrees to Radians/1

== system Last_version_po_STO/fourier_filter16 ==
  In1 : Inport
  Complex to Real-Imag1 : ComplexToRealImag
  Degrees to Radians : simulink_extras/Transformations/Degrees to Radians
  Fourier1 : powerlib_meascontrol/Measurements/Fourier  Freq=50  n=1  InInit=[0, 0]  Ts=0
      settings: SourceProductName=Simscape Electrical
  Gain1 : Gain  Gain=1/sqrt(2)
  Magnitude-Angle to Complex1 : MagnitudeAngleToComplex
  RMS : Outport
  Real : Outport  Port=2
  Imag : Outport  Port=3
  Complex : Outport  Port=4
  Phase : Outport  Port=5
  wires:
  Fourier1/2 -> Degrees to Radians/1
  In1/1 -> Fourier1/1
  Magnitude-Angle to Complex1/1 -> Complex/1, Complex to Real-Imag1/1
  Complex to Real-Imag1/2 -> Imag/1
  Complex to Real-Imag1/1 -> Real/1
  Degrees to Radians/1 -> Phase/1, Magnitude-Angle to Complex1/2
  Fourier1/1 -> Gain1/1
  Gain1/1 -> RMS/1, Magnitude-Angle to Complex1/1

== system Last_version_po_STO/fourier_filter17 ==
  In1 : Inport
  Complex to Real-Imag1 : ComplexToRealImag
  Degrees to Radians : simulink_extras/Transformations/Degrees to Radians
  Fourier1 : powerlib_meascontrol/Measurements/Fourier  Freq=50  n=1  InInit=[0, 0]  Ts=0
      settings: SourceProductName=Simscape Electrical
  Gain1 : Gain  Gain=1/sqrt(2)
  Magnitude-Angle to Complex1 : MagnitudeAngleToComplex
  RMS : Outport
  Real : Outport  Port=2
  Imag : Outport  Port=3
  Complex : Outport  Port=4
  Phase : Outport  Port=5
  wires:
  Gain1/1 -> Magnitude-Angle to Complex1/1, RMS/1
  Fourier1/1 -> Gain1/1
  Degrees to Radians/1 -> Magnitude-Angle to Complex1/2, Phase/1
  Complex to Real-Imag1/1 -> Real/1
  Complex to Real-Imag1/2 -> Imag/1
  Magnitude-Angle to Complex1/1 -> Complex to Real-Imag1/1, Complex/1
  In1/1 -> Fourier1/1
  Fourier1/2 -> Degrees to Radians/1

== system Last_version_po_STO/fourier_filter18 ==
  In1 : Inport
  Complex to Real-Imag1 : ComplexToRealImag
  Degrees to Radians : simulink_extras/Transformations/Degrees to Radians
  Fourier1 : powerlib_meascontrol/Measurements/Fourier  Freq=50  n=1  InInit=[0, 0]  Ts=0
      settings: SourceProductName=Simscape Electrical
  Gain1 : Gain  Gain=1/sqrt(2)
  Magnitude-Angle to Complex1 : MagnitudeAngleToComplex
  RMS : Outport
  Real : Outport  Port=2
  Imag : Outport  Port=3
  Complex : Outport  Port=4
  Phase : Outport  Port=5
  wires:
  Fourier1/2 -> Degrees to Radians/1
  In1/1 -> Fourier1/1
  Magnitude-Angle to Complex1/1 -> Complex/1, Complex to Real-Imag1/1
  Complex to Real-Imag1/2 -> Imag/1
  Complex to Real-Imag1/1 -> Real/1
  Degrees to Radians/1 -> Phase/1, Magnitude-Angle to Complex1/2
  Fourier1/1 -> Gain1/1
  Gain1/1 -> RMS/1, Magnitude-Angle to Complex1/1

== system Last_version_po_STO/fourier_filter19 ==
  In1 : Inport
  Complex to Real-Imag1 : ComplexToRealImag
  Degrees to Radians : simulink_extras/Transformations/Degrees to Radians
  Fourier1 : powerlib_meascontrol/Measurements/Fourier  Freq=50  n=1  InInit=[0, 0]  Ts=0
      settings: SourceProductName=Simscape Electrical
  Gain1 : Gain  Gain=1/sqrt(2)
  Magnitude-Angle to Complex1 : MagnitudeAngleToComplex
  RMS : Outport
  Real : Outport  Port=2
  Imag : Outport  Port=3
  Complex : Outport  Port=4
  Phase : Outport  Port=5
  wires:
  Gain1/1 -> Magnitude-Angle to Complex1/1, RMS/1
  Fourier1/1 -> Gain1/1
  Degrees to Radians/1 -> Magnitude-Angle to Complex1/2, Phase/1
  Complex to Real-Imag1/1 -> Real/1
  Complex to Real-Imag1/2 -> Imag/1
  Magnitude-Angle to Complex1/1 -> Complex to Real-Imag1/1, Complex/1
  In1/1 -> Fourier1/1
  Fourier1/2 -> Degrees to Radians/1

== system Last_version_po_STO/fourier_filter2 ==
  In1 : Inport
  Complex to Real-Imag1 : ComplexToRealImag
  Degrees to Radians : simulink_extras/Transformations/Degrees to Radians
  Fourier1 : powerlib_meascontrol/Measurements/Fourier  Freq=50  n=1  InInit=[0, 0]  Ts=0
      settings: SourceProductName=Simscape Electrical
  Gain1 : Gain  Gain=1/sqrt(2)
  Magnitude-Angle to Complex1 : MagnitudeAngleToComplex
  RMS : Outport
  Real : Outport  Port=2
  Imag : Outport  Port=3
  Complex : Outport  Port=4
  Phase : Outport  Port=5
  wires:
  Fourier1/2 -> Degrees to Radians/1
  In1/1 -> Fourier1/1
  Magnitude-Angle to Complex1/1 -> Complex/1, Complex to Real-Imag1/1
  Complex to Real-Imag1/2 -> Imag/1
  Complex to Real-Imag1/1 -> Real/1
  Degrees to Radians/1 -> Phase/1, Magnitude-Angle to Complex1/2
  Fourier1/1 -> Gain1/1
  Gain1/1 -> RMS/1, Magnitude-Angle to Complex1/1
